simulink model "DroneModelv6"  (R2023b)
settings: Solver=VariableStepAuto  StartTime=0.0  StopTime=1  RelTol=1e-3
undefined symbols (not defined in the file): bref, mass, stab_CFx, stab_CFy, stab_CFz, stab_CMx, stab_CMy, stab_CMz, wing_CFx, wing_CFy, wing_CFz, wing_CMx, wing_CMy, wing_CMz, x_cg, y_cg, z_cg
libraries: aerolibasang x3, slpidlib x2, aerolibconvert2 x2, shared6dof x1, aerolibadyn x1, aerolibatmos2 x1
settings Model: SimulationMode=accelerator  Creator=Avery  LastModifiedBy=Avery
settings OptimizationCC: BlockReduction=off  ConditionallyExecuteInputs=off

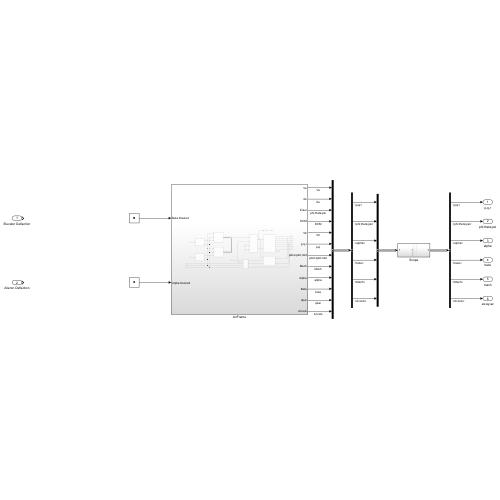
[thumbnail: Simulink's stored preview of the top-level diagram]
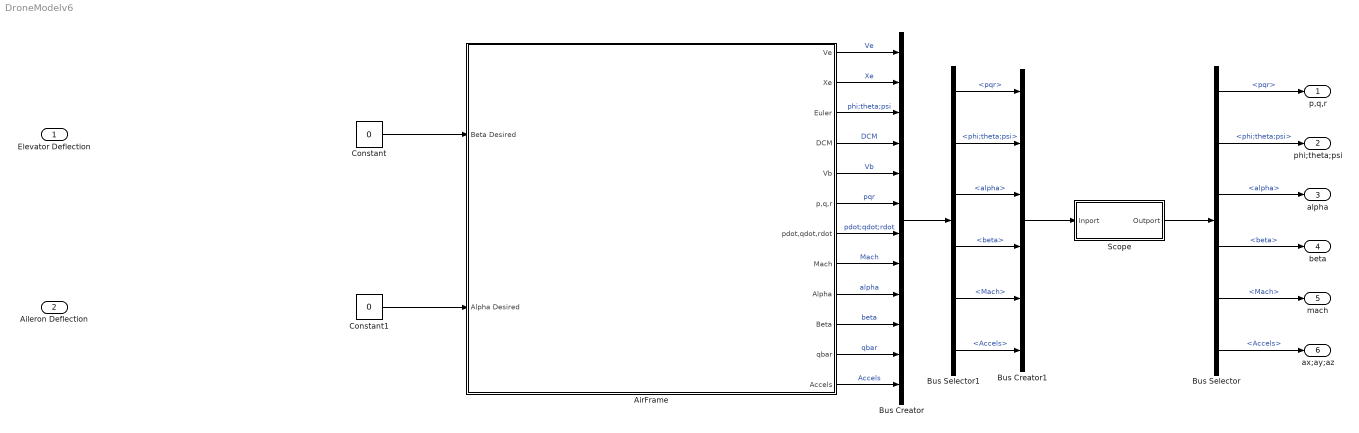
== system DroneModelv6 ==
  Elevator Deflection : Inport
  Aileron Deflection : Inport  Port=2
  AirFrame : Subsystem
  Bus Creator : BusCreator  Inputs=12
  Bus Creator1 : BusCreator  Inputs=6
  Bus Selector : BusSelector  OutputSignals=pqr,phi;theta;psi,alpha,beta,Mach,Accels
  Bus Selector1 : BusSelector  OutputSignals=pqr,phi;theta;psi,alpha,beta,Mach,Accels
  Constant : Constant  Value=0
  Constant1 : Constant  Value=0
  Scope : Subsystem
  p,q,r : Outport
  phi;theta;psi : Outport  Port=2
  alpha : Outport  Port=3
  beta : Outport  Port=4
  mach : Outport  Port=5
  ax;ay;az : Outport  Port=6
  wires:
  AirFrame/12(Accels) -> Bus Creator/12  "Accels"
  AirFrame/11(qbar) -> Bus Creator/11  "qbar"
  AirFrame/10(Beta) -> Bus Creator/10  "beta"
  AirFrame/9(Alpha) -> Bus Creator/9  "alpha"
  AirFrame/8(Mach) -> Bus Creator/8  "Mach"
  AirFrame/7(pdot,qdot,rdot) -> Bus Creator/7  "pdot;qdot;rdot"
  AirFrame/6(p,q,r) -> Bus Creator/6  "pqr"
  AirFrame/5(Vb) -> Bus Creator/5  "Vb"
  AirFrame/4(DCM) -> Bus Creator/4  "DCM"
  AirFrame/3(Euler) -> Bus Creator/3  "phi;theta;psi"
  AirFrame/2(Xe) -> Bus Creator/2  "Xe"
  AirFrame/1(Ve) -> Bus Creator/1  "Ve"
  Bus Creator1/1 -> Scope/1(Inport)
  Bus Creator/1 -> Bus Selector1/1
  Scope/1(Outport) -> Bus Selector/1
  Bus Selector/1 -> p,q,r/1  "<pqr>"
  Bus Selector/2 -> phi;theta;psi/1  "<phi;theta;psi>"
  Bus Selector/3 -> alpha/1  "<alpha>"
  Bus Selector/4 -> beta/1  "<beta>"
  Bus Selector/5 -> mach/1  "<Mach>"
  Bus Selector/6 -> ax;ay;az/1  "<Accels>"
  Bus Selector1/1 -> Bus Creator1/1  "<pqr>"
  Bus Selector1/2 -> Bus Creator1/2  "<phi;theta;psi>"
  Bus Selector1/3 -> Bus Creator1/3  "<alpha>"
  Bus Selector1/4 -> Bus Creator1/4  "<beta>"
  Bus Selector1/5 -> Bus Creator1/5  "<Mach>"
  Bus Selector1/6 -> Bus Creator1/6  "<Accels>"
  Constant/1 -> AirFrame/1(Beta Desired)
  Constant1/1 -> AirFrame/2(Alpha Desired)

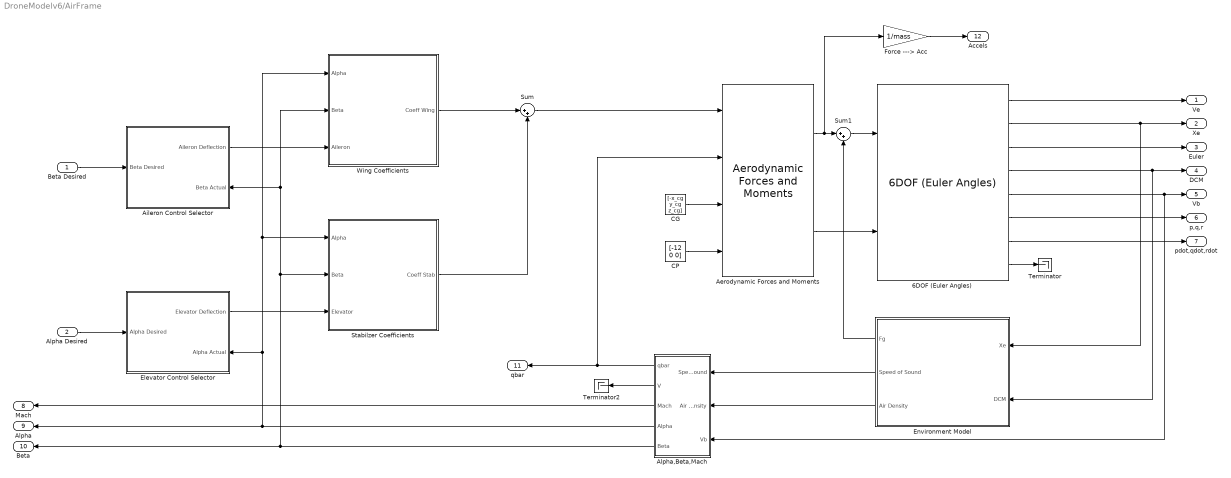
== system DroneModelv6/AirFrame ==
  Beta Desired : Inport
  Alpha Desired : Inport  Port=2
  6DOF (Euler Angles) : shared6dof/6DOF (Euler Angles)  units=Metric (MKS)  mtype=Fixed  rep=Quaternion  xme_0=init_pos_inertial  Vm_0=init_velo_body  eul_0=init_euler_orien  pm_0=init_body_rot  mass_0=mass  mass_e=0.5  mass_f=2.0  inertia=init_inertia  inertia_e=eye(3)  inertia_f=2*eye(3)  k_quat=1.0  vre_flag=on  abi_flag=off  aMode=0  xme_statename=''  Vm_statename=''  eul_statename=''  quat_statename=''  pm_statename=''  mass_statename=''
  "Aerodynamic Forces and Moments " : aerolibadyn/Aerodynamic Forces and Moments   inputAxes=Body  outputForceAxes=Body  outputMomentAxes=Body  S=Sref  b=bref  cbar=cref
  Aileron Control Selector : Subsystem
      settings: PortSchema="{\"entries\":[{\"content\":{\"sides\":[{\"content\":{\"connectorIds\":[\"In1\"]},\"type\":\"ConnectorPlacement.EquallySpacedRectSide\",\"uuid\":\"3692c7d6-6772-4b92-819a-cef574290569\"},{\"content\":{\"connectorIds\":[\"Out1\",\"In2\"],\"side\":\"RIGHT\"},\"type\":\"ConnectorPlacement.EquallySpacedRectSide\",\"uuid\":\"905d3b98-0635-4eca-960c-e0840bd01458\"},{\"content\":{\"side\":\"TOP\"},\"type\":\"ConnectorPlacement.EquallySpacedRectSide\",\"uuid\":\"5dcf80d0-43aa-4186-ba58-6be542882c64\"}]},\"type\":\"ConnectorPlacement.EquallySpacedConnector\",\"uuid\":\"ac153307-cb0b-4869-8145-be6cdbdfec88\"}],\"packageUris\":[\"http://schema.mathworks.com/mf0/Connector/R2020b\"],\"version\":\"1.0\"}"
  Alpha,Beta,Mach : Subsystem
  CG : Constant  Value=[-x_cg y_cg z_cg]
  CP : Constant  Value=[-12 0 0]
  Elevator Control Selector : Subsystem
      settings: PortSchema="{\"entries\":[{\"content\":{\"sides\":[{\"content\":{\"connectorIds\":[\"In1\"]},\"type\":\"ConnectorPlacement.EquallySpacedRectSide\",\"uuid\":\"bce9c69c-277c-4e2d-b000-96b998c6b0ec\"},{\"content\":{\"connectorIds\":[\"Out1\",\"In2\"],\"side\":\"RIGHT\"},\"type\":\"ConnectorPlacement.EquallySpacedRectSide\",\"uuid\":\"b73180a2-921e-4245-83cf-65a8a701d2fc\"},{\"content\":{\"side\":\"TOP\"},\"type\":\"ConnectorPlacement.EquallySpacedRectSide\",\"uuid\":\"a7d610d5-990d-4f96-b8aa-182502f54a5a\"}]},\"type\":\"ConnectorPlacement.EquallySpacedConnector\",\"uuid\":\"40862d1a-860a-4139-a354-3400513bb2f3\"}],\"packageUris\":[\"http://schema.mathworks.com/mf0/Connector/R2020b\"],\"version\":\"1.0\"}"
  Environment Model : Subsystem
  Force ---> Acc : Gain  Gain=1/mass  SaturateOnIntegerOverflow=on  OutDataTypeStr=Inherit: Same as input  ParamDataTypeStr=Inherit: Same as input
  Stabilzer Coefficients : Subsystem
  Sum : Sum  Inputs=|++
  Sum1 : Sum  Inputs=|++
  Terminator : Terminator
  Terminator2 : Terminator
  Wing Coefficients : Subsystem
  Ve : Outport
  Xe : Outport  Port=2
  Euler : Outport  Port=3
  DCM : Outport  Port=4
  Vb : Outport  Port=5
  p,q,r : Outport  Port=6
  pdot,qdot,rdot : Outport  Port=7
  Mach : Outport  Port=8
  Alpha : Outport  Port=9
  Beta : Outport  Port=10
  qbar : Outport  Port=11
  Accels : Outport  Port=12
  wires:
  Environment Model/3(Air Density) -> Alpha,Beta,Mach/2(Air Density)
  6DOF (Euler Angles)/6 -> p,q,r/1
  6DOF (Euler Angles)/4 -> DCM/1, Environment Model/2(DCM)
  6DOF (Euler Angles)/2 -> Xe/1, Environment Model/1(Xe)
  6DOF (Euler Angles)/5 -> Vb/1, Alpha,Beta,Mach/3(Vb)
  "Aerodynamic Forces and Moments "/1 -> Force ---> Acc/1, Sum1/1
  6DOF (Euler Angles)/3 -> Euler/1
  Wing Coefficients/1(Coeff Wing) -> Sum/1
  6DOF (Euler Angles)/1 -> Ve/1
  CP/1 -> "Aerodynamic Forces and Moments "/4
  Stabilzer Coefficients/1(Coeff Stab) -> Sum/2
  Alpha,Beta,Mach/1(qbar) -> qbar/1, "Aerodynamic Forces and Moments "/2
  CG/1 -> "Aerodynamic Forces and Moments "/3
  Alpha,Beta,Mach/4(Alpha) -> Alpha/1, Elevator Control Selector/2(Alpha Actual), Stabilzer Coefficients/1(Alpha), Wing Coefficients/1(Alpha)
  6DOF (Euler Angles)/8 -> Terminator/1
  "Aerodynamic Forces and Moments "/2 -> 6DOF (Euler Angles)/2
  6DOF (Euler Angles)/7 -> pdot,qdot,rdot/1
  Alpha,Beta,Mach/2(V) -> Terminator2/1
  Environment Model/1(Fg) -> Sum1/2
  Environment Model/2(Speed of Sound) -> Alpha,Beta,Mach/1(Speed of Sound)
  Sum/1 -> "Aerodynamic Forces and Moments "/1
  Sum1/1 -> 6DOF (Euler Angles)/1
  Force ---> Acc/1 -> Accels/1
  Aileron Control Selector/1(Aileron Deflection) -> Wing Coefficients/3(Aileron)
  Alpha,Beta,Mach/5(Beta) -> Beta/1, Wing Coefficients/2(Beta), Aileron Control Selector/2(Beta Actual), Stabilzer Coefficients/2(Beta)
  Beta Desired/1 -> Aileron Control Selector/1(Beta Desired)
  Elevator Control Selector/1(Elevator Deflection) -> Stabilzer Coefficients/3(Elevator)
  Alpha Desired/1 -> Elevator Control Selector/1(Alpha Desired)
  Alpha,Beta,Mach/3(Mach) -> Mach/1

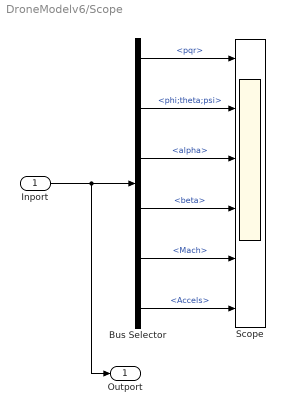
== system DroneModelv6/Scope ==
  Inport : Inport
  Bus Selector : BusSelector  OutputSignals=pqr,phi;theta;psi,alpha,beta,Mach,Accels
  Scope : Scope  NumInputPorts=6
  Outport : Outport
  wires:
  Inport/1 -> Outport/1, Bus Selector/1
  Bus Selector/6 -> Scope/6  "<Accels>"
  Bus Selector/5 -> Scope/5  "<Mach>"
  Bus Selector/4 -> Scope/4  "<beta>"
  Bus Selector/3 -> Scope/3  "<alpha>"
  Bus Selector/2 -> Scope/2  "<phi;theta;psi>"
  Bus Selector/1 -> Scope/1  "<pqr>"

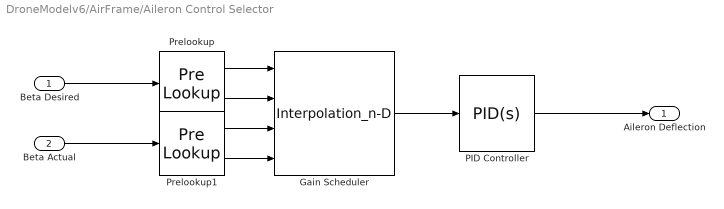
== system DroneModelv6/AirFrame/Aileron Control Selector ==
  Beta Desired : Inport
  Beta Actual : Inport  Port=2
  Gain Scheduler : Interpolation_n-D  InternalRulePriority=Speed
  PID Controller : slpidlib/PID Controller  Controller=PID  Form=Parallel  TimeDomain=Continuous-time  UseExternalTs=off  SampleTime=-1  IntegratorMethod=Forward Euler  FilterMethod=Forward Euler  ControllerParametersSource=internal  P=1  I=1  UseKiTs=off  D=0  N=100  UseFilter=on  TunerSelectOption=Transfer Function Based (PID Tuner App)  InitialConditionSource=internal  InitialConditionForIntegrator=0  InitialConditionForFilter=0  DifferentiatorICPrevScaledInput=0  ExternalReset=none  TrackingMode=off  Kt=1  LimitOutput=off  SatLimitsSource=internal  UpperSaturationLimit=inf  LowerSaturationLimit=-inf  LinearizeAsGain=on  AntiWindupMode=none  Kb=1  LimitIntegrator=off  UpperIntegratorSaturationLimit=inf  LowerIntegratorSaturationLimit=-inf  POutMin=[]  POutMax=[]  IOutMin=[]  IOutMax=[]  DOutMin=[]  DOutMax=[]  NOutMin=[]  NOutMax=[]  SumOutMin=[]  SumOutMax=[]  SaturationOutMin=[]  SaturationOutMax=[]  PParamMin=[]  PParamMax=[]  IParamMin=[]  IParamMax=[]  DParamMin=[]  DParamMax=[]  NParamMin=[]  NParamMax=[]  KbParamMin=[]  KbParamMax=[]  KtParamMin=[]  KtParamMax=[]  KbOutMin=[]  KbOutMax=[]  KtOutMin=[]  KtOutMax=[]  IntegratorOutMin=[]  IntegratorOutMax=[]  FilterOutMin=[]  FilterOutMax=[]  SumI1OutMin=[]  SumI1OutMax=[]  SumI2OutMin=[]  SumI2OutMax=[]  SumI3OutMin=[]  SumI3OutMax=[]  SumI4OutMin=[]  SumI4OutMax=[]  SumDOutMin=[]  SumDOutMax=[]  DifferentiatorOutMin=[]  DifferentiatorOutMax=[]  FilterDiffOutCoefMin=[]  FilterDiffOutCoefMax=[]  ReciprocalOutMin=[]  ReciprocalOutMax=[]  SumDenOutMin=[]  SumDenOutMax=[]  SumNumOutMin=[]  SumNumOutMax=[]  DivideOutMin=[]  DivideOutMax=[]  UdiffTsProdOutMin=[]  UdiffTsProdOutMax=[]  NTsProdOutMin=[]  NTsProdOutMax=[]  UintegralTsProdOutMin=[]  UintegralTsProdOutMax=[]  UngainTsProdOutMin=[]  UngainTsProdOutMax=[]  ClampingZeroOutDataTypeStr=Inherit: Inherit via back propagation  ClampingZeroOutMin=[]  ClampingZeroOutMax=[]  FilterDenConstantOutDataTypeStr=Inherit: Inherit via back propagation  FilterDenConstantOutMin=[]  FilterDenConstantOutMax=[]  PCopyOutDataTypeStr=Inherit: Inherit via back propagation  PCopyOutMin=[]  PCopyOutMax=[]  NCopyOutDataTypeStr=Inherit: Inherit via back propagation  NCopyOutMin=[]  NCopyOutMax=[]  IntegratorContinuousStateAttributes=''  IntegratorStateMustResolveToSignalObject=off  IntegratorRTWStateStorageClass=Auto  FilterContinuousStateAttributes=''  FilterStateMustResolveToSignalObject=off  FilterRTWStateStorageClass=Auto  ParallelPVariant=InternalParameters  IdealPVariant=Disabled  IVariant=InternalParameters  DVariant=InternalParameters  IntegratorVariant=Continuous  SatVariant=Disabled  AWVariant=Passthrough  PCopyVariant=Disabled  TRVariant=Disabled  FdbkBlocksVariant=Forward  IdealPFdbkVariant=Disabled  SatFdbkVariant=Disabled  DerivativeFilterVariant=ContFilter  NVariant=InternalParameters  NCopyVariant=Disabled  FilterICVariant=InternalICsFilter  IntegratorICVariant=InternalICs  ExternalResetVariant=Disabled  TRSumVariant=Passthrough  SumFdbkVariant=Disabled  SumVariant=Sum_PID  TsampFilterVariant=InternalTs  TsampNgainVariant=Passthrough  TsampIntegralVariant=Disabled_SignalSpec  ExternalSaturationOutDataTypeStr=Inherit: Same as second input
  Prelookup : PreLookup  BreakpointsData=[10:10:110]  ExtrapMethod=Linear
  Prelookup1 : PreLookup  BreakpointsData=[10:10:110]  ExtrapMethod=Linear
  Aileron Deflection : Outport
  wires:
  Prelookup1/2 -> Gain Scheduler/4
  Prelookup1/1 -> Gain Scheduler/3
  Prelookup/2 -> Gain Scheduler/2
  Prelookup/1 -> Gain Scheduler/1
  Beta Desired/1 -> Prelookup/1
  Beta Actual/1 -> Prelookup1/1
  Gain Scheduler/1 -> PID Controller/1
  PID Controller/1 -> Aileron Deflection/1

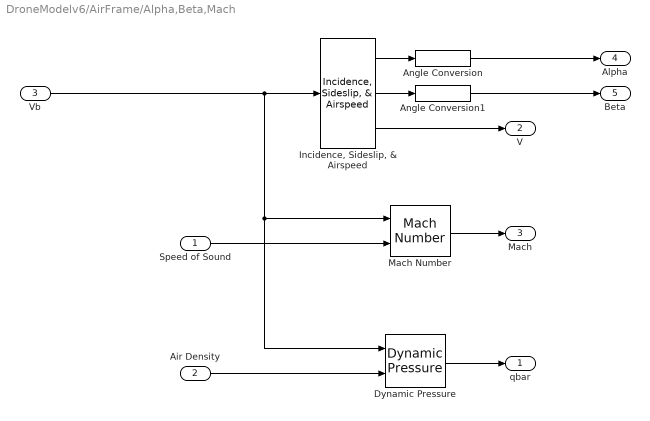
== system DroneModelv6/AirFrame/Alpha,Beta,Mach ==
  Speed of Sound : Inport
  Air Density : Inport  Port=2
  Vb : Inport  Port=3
  Angle Conversion : aerolibconvert2/Angle Conversion  IU=rad  OU=deg
  Angle Conversion1 : aerolibconvert2/Angle Conversion  IU=rad  OU=deg
  Dynamic Pressure : aerolibasang/Dynamic Pressure
  "Incidence, Sideslip, & Airspeed" : aerolibasang/Incidence, Sideslip, & Airspeed
  Mach Number : aerolibasang/Mach Number
  qbar : Outport
  V : Outport  Port=2
  Mach : Outport  Port=3
  Alpha : Outport  Port=4
  Beta : Outport  Port=5
  wires:
  "Incidence, Sideslip, & Airspeed"/3 -> V/1
  "Incidence, Sideslip, & Airspeed"/2 -> Angle Conversion1/1
  "Incidence, Sideslip, & Airspeed"/1 -> Angle Conversion/1
  Speed of Sound/1 -> Mach Number/2
  Mach Number/1 -> Mach/1
  Air Density/1 -> Dynamic Pressure/2
  Dynamic Pressure/1 -> qbar/1
  Angle Conversion/1 -> Alpha/1
  Vb/1 -> Dynamic Pressure/1, Mach Number/1, "Incidence, Sideslip, & Airspeed"/1
  Angle Conversion1/1 -> Beta/1

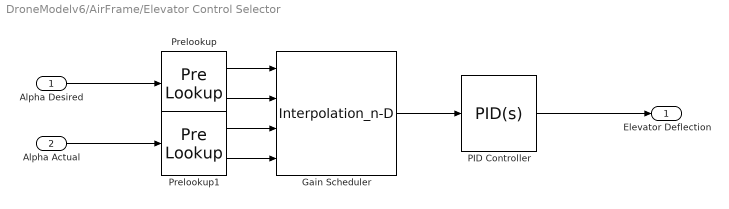
== system DroneModelv6/AirFrame/Elevator Control Selector ==
  Alpha Desired : Inport
  Alpha Actual : Inport  Port=2
  Gain Scheduler : Interpolation_n-D  InternalRulePriority=Speed
  PID Controller : slpidlib/PID Controller  Controller=PID  Form=Parallel  TimeDomain=Continuous-time  UseExternalTs=off  SampleTime=-1  IntegratorMethod=Forward Euler  FilterMethod=Forward Euler  ControllerParametersSource=internal  P=1  I=1  UseKiTs=off  D=0  N=100  UseFilter=on  TunerSelectOption=Transfer Function Based (PID Tuner App)  InitialConditionSource=internal  InitialConditionForIntegrator=0  InitialConditionForFilter=0  DifferentiatorICPrevScaledInput=0  ExternalReset=none  TrackingMode=off  Kt=1  LimitOutput=off  SatLimitsSource=internal  UpperSaturationLimit=inf  LowerSaturationLimit=-inf  LinearizeAsGain=on  AntiWindupMode=none  Kb=1  LimitIntegrator=off  UpperIntegratorSaturationLimit=inf  LowerIntegratorSaturationLimit=-inf  POutMin=[]  POutMax=[]  IOutMin=[]  IOutMax=[]  DOutMin=[]  DOutMax=[]  NOutMin=[]  NOutMax=[]  SumOutMin=[]  SumOutMax=[]  SaturationOutMin=[]  SaturationOutMax=[]  PParamMin=[]  PParamMax=[]  IParamMin=[]  IParamMax=[]  DParamMin=[]  DParamMax=[]  NParamMin=[]  NParamMax=[]  KbParamMin=[]  KbParamMax=[]  KtParamMin=[]  KtParamMax=[]  KbOutMin=[]  KbOutMax=[]  KtOutMin=[]  KtOutMax=[]  IntegratorOutMin=[]  IntegratorOutMax=[]  FilterOutMin=[]  FilterOutMax=[]  SumI1OutMin=[]  SumI1OutMax=[]  SumI2OutMin=[]  SumI2OutMax=[]  SumI3OutMin=[]  SumI3OutMax=[]  SumI4OutMin=[]  SumI4OutMax=[]  SumDOutMin=[]  SumDOutMax=[]  DifferentiatorOutMin=[]  DifferentiatorOutMax=[]  FilterDiffOutCoefMin=[]  FilterDiffOutCoefMax=[]  ReciprocalOutMin=[]  ReciprocalOutMax=[]  SumDenOutMin=[]  SumDenOutMax=[]  SumNumOutMin=[]  SumNumOutMax=[]  DivideOutMin=[]  DivideOutMax=[]  UdiffTsProdOutMin=[]  UdiffTsProdOutMax=[]  NTsProdOutMin=[]  NTsProdOutMax=[]  UintegralTsProdOutMin=[]  UintegralTsProdOutMax=[]  UngainTsProdOutMin=[]  UngainTsProdOutMax=[]  ClampingZeroOutDataTypeStr=Inherit: Inherit via back propagation  ClampingZeroOutMin=[]  ClampingZeroOutMax=[]  FilterDenConstantOutDataTypeStr=Inherit: Inherit via back propagation  FilterDenConstantOutMin=[]  FilterDenConstantOutMax=[]  PCopyOutDataTypeStr=Inherit: Inherit via back propagation  PCopyOutMin=[]  PCopyOutMax=[]  NCopyOutDataTypeStr=Inherit: Inherit via back propagation  NCopyOutMin=[]  NCopyOutMax=[]  IntegratorContinuousStateAttributes=''  IntegratorStateMustResolveToSignalObject=off  IntegratorRTWStateStorageClass=Auto  FilterContinuousStateAttributes=''  FilterStateMustResolveToSignalObject=off  FilterRTWStateStorageClass=Auto  ParallelPVariant=InternalParameters  IdealPVariant=Disabled  IVariant=InternalParameters  DVariant=InternalParameters  IntegratorVariant=Continuous  SatVariant=Disabled  AWVariant=Passthrough  PCopyVariant=Disabled  TRVariant=Disabled  FdbkBlocksVariant=Forward  IdealPFdbkVariant=Disabled  SatFdbkVariant=Disabled  DerivativeFilterVariant=ContFilter  NVariant=InternalParameters  NCopyVariant=Disabled  FilterICVariant=InternalICsFilter  IntegratorICVariant=InternalICs  ExternalResetVariant=Disabled  TRSumVariant=Passthrough  SumFdbkVariant=Disabled  SumVariant=Sum_PID  TsampFilterVariant=InternalTs  TsampNgainVariant=Passthrough  TsampIntegralVariant=Disabled_SignalSpec  ExternalSaturationOutDataTypeStr=Inherit: Same as second input
  Prelookup : PreLookup  BreakpointsData=[10:10:110]  ExtrapMethod=Linear
  Prelookup1 : PreLookup  BreakpointsData=[10:10:110]  ExtrapMethod=Linear
  Elevator Deflection : Outport
  wires:
  Prelookup1/2 -> Gain Scheduler/4
  Prelookup1/1 -> Gain Scheduler/3
  Gain Scheduler/1 -> PID Controller/1
  Prelookup/1 -> Gain Scheduler/1
  Alpha Actual/1 -> Prelookup1/1
  Alpha Desired/1 -> Prelookup/1
  PID Controller/1 -> Elevator Deflection/1
  Prelookup/2 -> Gain Scheduler/2

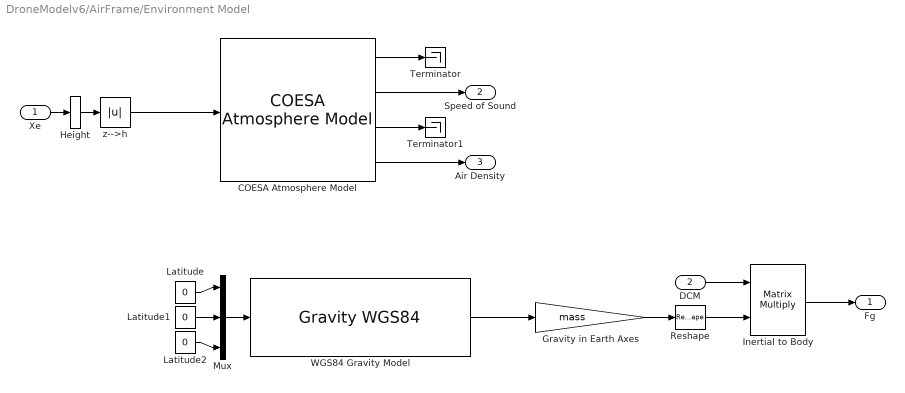
== system DroneModelv6/AirFrame/Environment Model ==
  Xe : Inport
  DCM : Inport  Port=2
  COESA Atmosphere Model : aerolibatmos2/COESA Atmosphere Model  units=Metric (MKS)  spec=1976 COESA-extended U.S. Standard Atmosphere  model=Profile  profile_var=High temperature  profile_percent=1%  profile_alt=5 km (16404 ft)  envelope_var=High temperature  envelope_percent=1%  action=Warning
  Gravity in Earth Axes : Gain  Gain=mass
  Height : Selector  InputPortWidth=3  IndexOptions=Index vector (dialog)  Indices=[3]  OutputSizes=1
  Inertial to Body : Product  Multiplication=Matrix(*)  InputSameDT=on  SaturateOnIntegerOverflow=on  OutDataTypeStr=Inherit: Same as first input
  Latitude : Constant  Value=0
  Latitude1 : Constant  Value=0
  Latitude2 : Constant  Value=0
  Mux : Mux  Inputs=3
  Reshape : Reshape
  Terminator : Terminator
  Terminator1 : Terminator
  "WGS84 Gravity Model  " : GravityWGS84
  z-->h : Abs
  Fg : Outport
  Speed of Sound : Outport  Port=2
  Air Density : Outport  Port=3
  wires:
  Height/1 -> z-->h/1
  Xe/1 -> Height/1
  COESA Atmosphere Model/1 -> Terminator/1
  COESA Atmosphere Model/3 -> Terminator1/1
  COESA Atmosphere Model/2 -> Speed of Sound/1
  COESA Atmosphere Model/4 -> Air Density/1
  "WGS84 Gravity Model  "/1 -> Gravity in Earth Axes/1
  Reshape/1 -> Inertial to Body/2
  Gravity in Earth Axes/1 -> Reshape/1
  DCM/1 -> Inertial to Body/1
  Inertial to Body/1 -> Fg/1
  Mux/1 -> "WGS84 Gravity Model  "/1
  Latitude/1 -> Mux/1
  Latitude1/1 -> Mux/2
  z-->h/1 -> COESA Atmosphere Model/1
  Latitude2/1 -> Mux/3

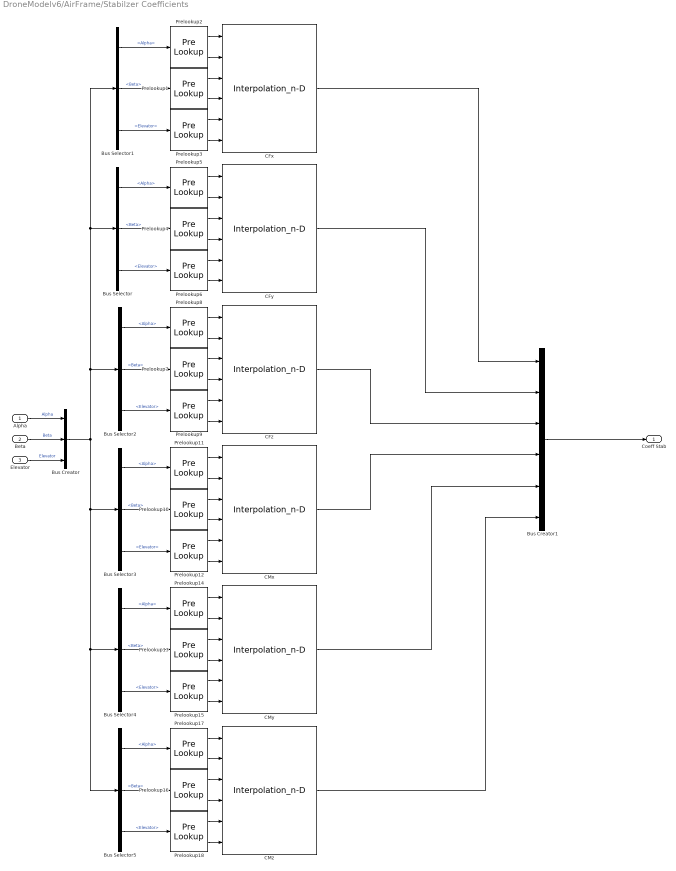
== system DroneModelv6/AirFrame/Stabilzer Coefficients ==
  Alpha : Inport
  Beta : Inport  Port=2
  Elevator : Inport  Port=3
  Bus Creator : BusCreator  Inputs=3
  Bus Creator1 : BusCreator  Inputs=6
  Bus Selector{,1..5} (6 alike) : BusSelector  OutputSignals=Alpha,Beta,Elevator
  CFx : Interpolation_n-D  NumberOfTableDimensions=3  Table=stab_CFx  InternalRulePriority=Speed
      settings: InputPortMap=u0,u1,u2,u3,u4,u5
  CFy : Interpolation_n-D  NumberOfTableDimensions=3  Table=stab_CFy  InternalRulePriority=Speed
      settings: InputPortMap=u0,u1,u2,u3,u4,u5
  CFz : Interpolation_n-D  NumberOfTableDimensions=3  Table=stab_CFz  InternalRulePriority=Speed
      settings: InputPortMap=u0,u1,u2,u3,u4,u5
  CMx : Interpolation_n-D  NumberOfTableDimensions=3  Table=stab_CMx  InternalRulePriority=Speed
      settings: InputPortMap=u0,u1,u2,u3,u4,u5
  CMy : Interpolation_n-D  NumberOfTableDimensions=3  Table=stab_CMy  InternalRulePriority=Speed
      settings: InputPortMap=u0,u1,u2,u3,u4,u5
  CMz : Interpolation_n-D  NumberOfTableDimensions=3  Table=stab_CMz  InternalRulePriority=Speed
      settings: InputPortMap=u0,u1,u2,u3,u4,u5
  Prelookup{1,4,7,10,13,16} (6 alike) : PreLookup  BreakpointsData=beta_val  ExtrapMethod=Linear
  Prelookup{2,5,8,11,14,17} (6 alike) : PreLookup  BreakpointsData=alpha_val  ExtrapMethod=Linear
  Prelookup{3,6,9,12,15,18} (6 alike) : PreLookup  BreakpointsData=elevator_val  ExtrapMethod=Linear
  Coeff Stab : Outport
  wires:
  Prelookup1/1 -> CFx/3
  Prelookup1/2 -> CFx/4
  Prelookup2/2 -> CFx/2
  Prelookup2/1 -> CFx/1
  Prelookup3/1 -> CFx/5
  Prelookup3/2 -> CFx/6
  Prelookup14/1 -> CMy/1
  Prelookup14/2 -> CMy/2
  Prelookup18/2 -> CMz/6
  Prelookup18/1 -> CMz/5
  Prelookup16/2 -> CMz/4
  Prelookup16/1 -> CMz/3
  Prelookup17/2 -> CMz/2
  Prelookup17/1 -> CMz/1
  Prelookup15/2 -> CMy/6
  Prelookup15/1 -> CMy/5
  Prelookup13/2 -> CMy/4
  Prelookup13/1 -> CMy/3
  Prelookup12/2 -> CMx/6
  Prelookup12/1 -> CMx/5
  Prelookup10/2 -> CMx/4
  Prelookup10/1 -> CMx/3
  Prelookup11/2 -> CMx/2
  Prelookup11/1 -> CMx/1
  Prelookup9/2 -> CFz/6
  Prelookup9/1 -> CFz/5
  Prelookup7/2 -> CFz/4
  Prelookup7/1 -> CFz/3
  Prelookup8/2 -> CFz/2
  Prelookup8/1 -> CFz/1
  Prelookup6/2 -> CFy/6
  Prelookup6/1 -> CFy/5
  Prelookup4/2 -> CFy/4
  Prelookup4/1 -> CFy/3
  Prelookup5/2 -> CFy/2
  Prelookup5/1 -> CFy/1
  Elevator/1 -> Bus Creator/3  "Elevator"
  Beta/1 -> Bus Creator/2  "Beta"
  Alpha/1 -> Bus Creator/1  "Alpha"
  Bus Selector1/3 -> Prelookup3/1  "<Elevator>"
  Bus Selector1/2 -> Prelookup1/1  "<Beta>"
  Bus Selector1/1 -> Prelookup2/1  "<Alpha>"
  Bus Selector/3 -> Prelookup6/1  "<Elevator>"
  Bus Selector/2 -> Prelookup4/1  "<Beta>"
  Bus Selector/1 -> Prelookup5/1  "<Alpha>"
  Bus Selector2/1 -> Prelookup8/1  "<Alpha>"
  Bus Selector2/2 -> Prelookup7/1  "<Beta>"
  Bus Selector2/3 -> Prelookup9/1  "<Elevator>"
  Bus Selector3/1 -> Prelookup11/1  "<Alpha>"
  Bus Selector3/2 -> Prelookup10/1  "<Beta>"
  Bus Selector3/3 -> Prelookup12/1  "<Elevator>"
  Bus Selector4/1 -> Prelookup14/1  "<Alpha>"
  Bus Selector4/2 -> Prelookup13/1  "<Beta>"
  Bus Selector4/3 -> Prelookup15/1  "<Elevator>"
  Bus Selector5/1 -> Prelookup17/1  "<Alpha>"
  Bus Selector5/2 -> Prelookup16/1  "<Beta>"
  Bus Selector5/3 -> Prelookup18/1  "<Elevator>"
  Bus Creator/1 -> Bus Selector1/1, Bus Selector/1, Bus Selector2/1, Bus Selector5/1, Bus Selector4/1, Bus Selector3/1
  CFx/1 -> Bus Creator1/1
  CFy/1 -> Bus Creator1/2
  CFz/1 -> Bus Creator1/3
  CMx/1 -> Bus Creator1/4
  CMy/1 -> Bus Creator1/5
  CMz/1 -> Bus Creator1/6
  Bus Creator1/1 -> Coeff Stab/1

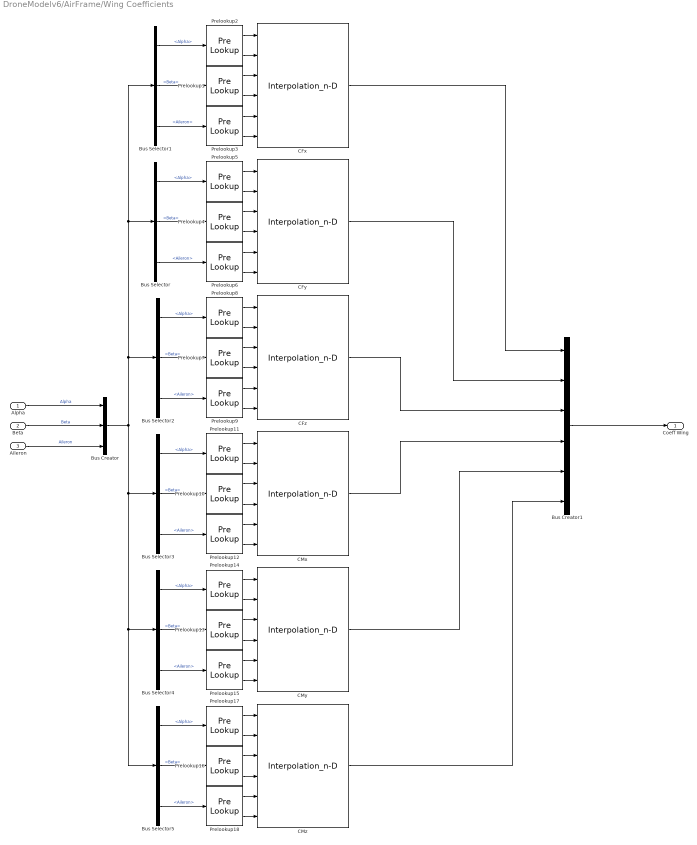
== system DroneModelv6/AirFrame/Wing Coefficients ==
  Alpha : Inport
  Beta : Inport  Port=2
  Aileron : Inport  Port=3
  Bus Creator : BusCreator  Inputs=3
  Bus Creator1 : BusCreator  Inputs=6
  Bus Selector{,1..5} (6 alike) : BusSelector  OutputSignals=Alpha,Beta,Aileron
  CFx : Interpolation_n-D  NumberOfTableDimensions=3  Table=wing_CFx  InternalRulePriority=Speed
      settings: InputPortMap=u0,u1,u2,u3,u4,u5
  CFy : Interpolation_n-D  NumberOfTableDimensions=3  Table=wing_CFy  InternalRulePriority=Speed
      settings: InputPortMap=u0,u1,u2,u3,u4,u5
  CFz : Interpolation_n-D  NumberOfTableDimensions=3  Table=wing_CFz  InternalRulePriority=Speed
      settings: InputPortMap=u0,u1,u2,u3,u4,u5
  CMx : Interpolation_n-D  NumberOfTableDimensions=3  Table=wing_CMx  InternalRulePriority=Speed
      settings: InputPortMap=u0,u1,u2,u3,u4,u5
  CMy : Interpolation_n-D  NumberOfTableDimensions=3  Table=wing_CMy  InternalRulePriority=Speed
      settings: InputPortMap=u0,u1,u2,u3,u4,u5
  CMz : Interpolation_n-D  NumberOfTableDimensions=3  Table=wing_CMz  InternalRulePriority=Speed
      settings: InputPortMap=u0,u1,u2,u3,u4,u5
  Prelookup{1,4,7,10,13,16} (6 alike) : PreLookup  BreakpointsData=beta_val  ExtrapMethod=Linear
  Prelookup{2,5,8,11,14,17} (6 alike) : PreLookup  BreakpointsData=alpha_val  ExtrapMethod=Linear
  Prelookup{3,6,9,12,15,18} (6 alike) : PreLookup  BreakpointsData=aileron_val  ExtrapMethod=Linear
  Coeff Wing : Outport
  wires:
  Prelookup1/1 -> CFx/3
  Prelookup1/2 -> CFx/4
  Prelookup2/2 -> CFx/2
  Prelookup2/1 -> CFx/1
  Prelookup3/1 -> CFx/5
  Prelookup3/2 -> CFx/6
  Prelookup14/1 -> CMy/1
  Prelookup14/2 -> CMy/2
  Prelookup18/2 -> CMz/6
  Prelookup18/1 -> CMz/5
  Prelookup16/2 -> CMz/4
  Prelookup16/1 -> CMz/3
  Prelookup17/2 -> CMz/2
  Prelookup17/1 -> CMz/1
  Prelookup15/2 -> CMy/6
  Prelookup15/1 -> CMy/5
  Prelookup13/2 -> CMy/4
  Prelookup13/1 -> CMy/3
  Prelookup12/2 -> CMx/6
  Prelookup12/1 -> CMx/5
  Prelookup10/2 -> CMx/4
  Prelookup10/1 -> CMx/3
  Prelookup11/2 -> CMx/2
  Prelookup11/1 -> CMx/1
  Prelookup9/2 -> CFz/6
  Prelookup9/1 -> CFz/5
  Prelookup7/2 -> CFz/4
  Prelookup7/1 -> CFz/3
  Prelookup8/2 -> CFz/2
  Prelookup8/1 -> CFz/1
  Prelookup6/2 -> CFy/6
  Prelookup6/1 -> CFy/5
  Prelookup4/2 -> CFy/4
  Prelookup4/1 -> CFy/3
  Prelookup5/2 -> CFy/2
  Prelookup5/1 -> CFy/1
  Aileron/1 -> Bus Creator/3  "Aileron"
  Beta/1 -> Bus Creator/2  "Beta"
  Alpha/1 -> Bus Creator/1  "Alpha"
  Bus Selector1/3 -> Prelookup3/1  "<Aileron>"
  Bus Selector1/2 -> Prelookup1/1  "<Beta>"
  Bus Selector1/1 -> Prelookup2/1  "<Alpha>"
  Bus Selector/3 -> Prelookup6/1  "<Aileron>"
  Bus Selector/2 -> Prelookup4/1  "<Beta>"
  Bus Selector/1 -> Prelookup5/1  "<Alpha>"
  Bus Selector2/1 -> Prelookup8/1  "<Alpha>"
  Bus Selector2/2 -> Prelookup7/1  "<Beta>"
  Bus Selector2/3 -> Prelookup9/1  "<Aileron>"
  Bus Selector3/1 -> Prelookup11/1  "<Alpha>"
  Bus Selector3/2 -> Prelookup10/1  "<Beta>"
  Bus Selector3/3 -> Prelookup12/1  "<Aileron>"
  Bus Selector4/1 -> Prelookup14/1  "<Alpha>"
  Bus Selector4/2 -> Prelookup13/1  "<Beta>"
  Bus Selector4/3 -> Prelookup15/1  "<Aileron>"
  Bus Selector5/1 -> Prelookup17/1  "<Alpha>"
  Bus Selector5/2 -> Prelookup16/1  "<Beta>"
  Bus Selector5/3 -> Prelookup18/1  "<Aileron>"
  Bus Creator/1 -> Bus Selector1/1, Bus Selector/1, Bus Selector2/1, Bus Selector5/1, Bus Selector4/1, Bus Selector3/1
  CFx/1 -> Bus Creator1/1
  CFy/1 -> Bus Creator1/2
  CFz/1 -> Bus Creator1/3
  CMx/1 -> Bus Creator1/4
  CMy/1 -> Bus Creator1/5
  CMz/1 -> Bus Creator1/6
  Bus Creator1/1 -> Coeff Wing/1
